simulink model "gstut14"  (Simulink 5.0)
settings: Solver=FixedStepDiscrete  StartTime=0.0  StopTime=0.5  RelTol=1e-3
undefined symbols (not defined in the file or in its folder): get, jet
libraries: dspbuff3 x2, dspsnks4 x2, dspspect3 x1, dspsrcs4 x1, dspmtrx3 x1, dspmathops x1
settings Model: LastModifiedBy=cclarke  SignalLoggingName=logsOut  ConditionalExecOptimization=on  ZeroCrossControl=UseLocalSettings  RTWMathFcnLibMatFile=iso_c_tmw.mat  RTWOptions="-aEnforceIntegerDowncast=1 -aFoldNonRolledExpr=1 -aInlineInvariantSignals=1 -aInlineParameters=0 -aLocalBlockOutputs=1 -aRollThreshold=5 -aRTWVerbose=1 -aGenerateReport=0 -aForceParamTrailComments=0 -aGenerateComments=1 -aIgnoreCustomStorageClasses=1 -aIncHierarchyInIds=0 -aMaxRTWIdLen=31 -aShowEliminatedStatements=0 -aReadOnly=0 -aIncDataTypeInIds=0 -aPrefixModelToSubsysFcnNames=1 -aInlinedPrmAccess=\"Literals\" -aGenerateFullHeader=1 -aIsPILTarget=0 -aLogVarNameModifier=\"rt_\" -aExtMode=0 -aExtModeTesting=0 -aExtModeTransport=\"tcpip\"  -aInlineParameters=0"

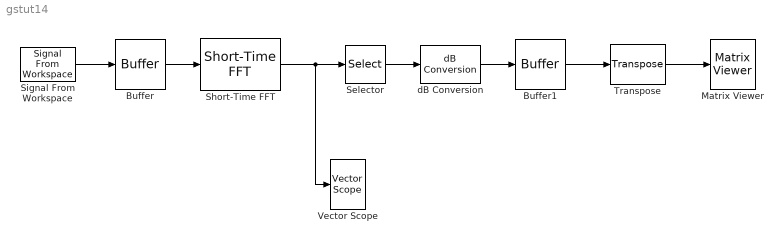
== system gstut14 ==
  Buffer : dspbuff3/Buffer  N=128  V=48  ic=0
  Buffer1 : dspbuff3/Buffer  N=48  V=46  ic=-70
  Matrix Viewer : dspsnks4/Matrix Viewer  ImageParams=on  CMapStr=jet(256)  AxisColorbar=on  AxisParams=on  AxisOrigin=Lower left corner  XLabel=Time Index  YLabel=Frequency Index  ZLabel=dB Magnitude  FigPos=get(0,'defaultfigureposition')  AxisZoom=off
      settings: YMin=-70  YMax=15
  Selector : Selector  Elements=1:64  InputPortWidth=128
  Short-Time FFT : dspspect3/Short-Time FFT  wintype=Hamming  Rs=50  beta=5  winsamp=Periodic  inheritFFT=on  fftsize=256  navg=2
  Signal From Workspace : dspsrcs4/Signal From Workspace  X=mtlb  Ts=1/8000  nsamps=80  OutputAfterFinalValue=Setting to zero
  Transpose : dspmtrx3/Transpose  Hermitian=off
  Vector Scope : dspsnks4/Vector Scope  ScopeProperties=off  Domain=Frequency  HorizSpan=1  DisplayProperties=off  AxisGrid=on  Memory=off  FrameNumber=on  AxisLegend=off  AxisZoom=off  OpenScopeAtSimStart=on  OpenScopeImmediately=off  FigPos=get(0,'defaultfigureposition')  AxisProperties=off  XUnits=Hertz  XRange=[0...Fs/2]  InheritXIncr=on  XIncr=1  XLabel=Time  YUnits=dB  YLabel=Magnitude, dB  LineProperties=on
      settings: YMin=-49.3106585941378  YMax=5.11522162658351
  dB Conversion : dspmathops/dB Conversion  dBtype=dB  intype=Amplitude  R=1  fuzz=on
  wires:
  Signal From Workspace/1 -> Buffer/1
  Buffer/1 -> Short-Time FFT/1
  Short-Time FFT/1 -> Vector Scope/1, Selector/1
  Selector/1 -> dB Conversion/1
  dB Conversion/1 -> Buffer1/1
  Transpose/1 -> Matrix Viewer/1
  Buffer1/1 -> Transpose/1
